simulink model "loop_ctl_flex_test"  (R2019b)
settings: Solver=FixedStepDiscrete  StartTime=0.0  StopTime=400  RelTol=1e-3
libraries: simulink x1, lib_dsphdlcontrol_v1 x1
settings Model: DataTypeOverride=Off  Creator=mbabst  LastModifiedBy=mbabst
settings DataIOCC: SaveOutput=off  SaveTime=off  ReturnWorkspaceOutputs=off
settings OptimizationCC: BlockReduction=off  ConditionallyExecuteInputs=off  DefaultParameterBehavior=Inlined  LifeSpan=inf
settings DebuggingCC: AlgebraicLoopMsg=error  SingleTaskRateTransMsg=error  StrictBusMsg=ErrorOnBusTreatedAsVector  SFUnexpectedBacktrackingDiag=warning  SFNoUnconditionalDefaultTransitionDiag=warning  SFExecutionAtInitializationDiag=none  ArithmeticOperatorsInVariantConditions=warning
settings HardwareCC: ProdBitPerPointer=32  ProdBitPerSizeT=32  ProdBitPerPtrDiffT=32  ProdLargestAtomicFloat=None  ProdIntDivRoundTo=Undefined  ProdEndianess=Unspecified  ProdWordSize=32  ProdHWDeviceType=ASIC/FPGA->ASIC/FPGA  ProdEqTarget=off
settings SFSimCC: SimUseLocalCustomCode=off  CustomCodeUndefinedFunction=UseInterfaceOnly
settings RTWCC: RTWUseLocalCustomCode=off
settings CodeAppCC: StateflowObjectComments=on
settings GRTTargetCC: TargetLangStandard=C89/C90 (ANSI)
settings ConfigComp: CovMetricSettings=dw  CovHtmlReporting=on  CovSaveCumulativeToWorkspaceVar=on  CovSaveSingleToWorkspaceVar=on  CovExternalEMLEnable=off

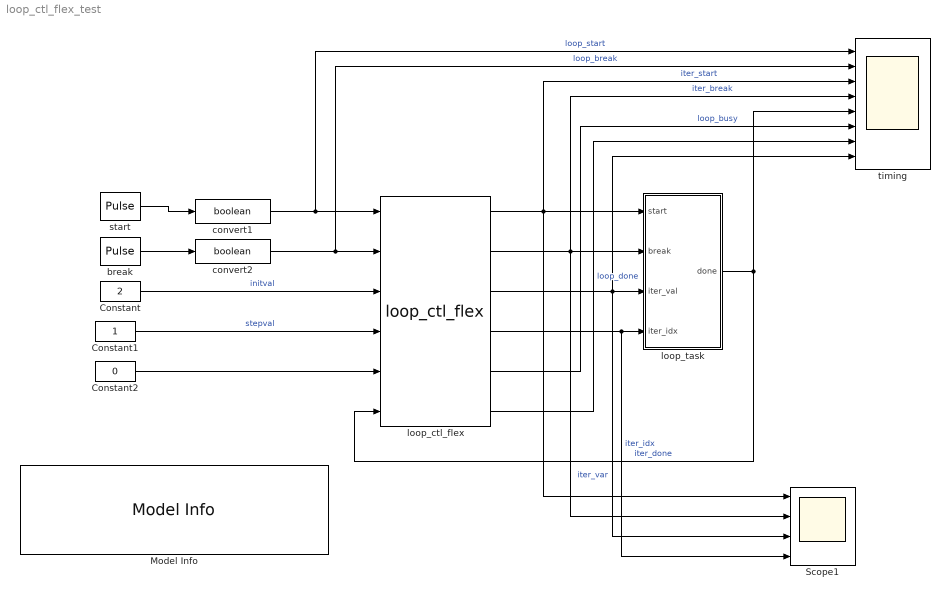
== system loop_ctl_flex_test ==
  Constant : Constant  Value=2  OutDataTypeStr=fixdt(1,8,4)  SampleTime=1
  Constant1 : Constant  OutDataTypeStr=fixdt(1,8,4)  SampleTime=1
  Constant2 : Constant  Value=0  OutDataTypeStr=fixdt(0,3,0)  SampleTime=1
  Model Info : simulink/Model-Wide Utilities/Model Info  Frame=on  DisplayStringWithTags=|  HorizontalTextAlignment=Left  LeftAlignmentValue=0.02
      | Copyright (c) 2005-2021 DSPlogic, Inc.
      | Distributed under the terms of the Simplified BSD License.
      | The full license is in the file LICENSE, distributed with this software.
      | 
      | Model: %<ModelName> (v%<ModelVersion>)
      | Author: Michael Babst <mike.babst@dsplogic.com>
      | Created: by %<Creator> on %<Created>
      | Modified: by %<ModifiedBy> on %<LastModificationDate>
  Scope1 : Scope  NumInputPorts=4
  break : DiscretePulseGenerator  Period=200  PhaseDelay=106
  convert1 : DataTypeConversion  OutDataTypeStr=boolean
  convert2 : DataTypeConversion  OutDataTypeStr=boolean
  loop_ctl_flex : lib_dsphdlcontrol_v1/loop_ctl_flex
      settings: SourceProductName=DSPHDL Library
  loop_task : Subsystem
  start : DiscretePulseGenerator  Period=100  PhaseDelay=5
  timing : Scope  NumInputPorts=8
  wires:
  start/1 -> convert1/1
  Constant/1 -> loop_ctl_flex/3  "initval"
  Constant1/1 -> loop_ctl_flex/4  "stepval"
  loop_task/1(done) -> timing/5, loop_ctl_flex/6  "iter_done"
  convert1/1 -> loop_ctl_flex/1, timing/1  "loop_start"
  Constant2/1 -> loop_ctl_flex/5
  break/1 -> convert2/1
  convert2/1 -> timing/2, loop_ctl_flex/2  "loop_break"
  loop_ctl_flex/2 -> loop_task/2(break), Scope1/2, timing/4  "iter_break"
  loop_ctl_flex/1 -> Scope1/1, timing/3, loop_task/1(start)  "iter_start"
  loop_ctl_flex/3 -> Scope1/3, timing/8, loop_task/3(iter_val)  "iter_var"
  loop_ctl_flex/4 -> Scope1/4, loop_task/4(iter_idx)  "iter_idx"
  loop_ctl_flex/5 -> timing/6  "loop_busy"
  loop_ctl_flex/6 -> timing/7  "loop_done"

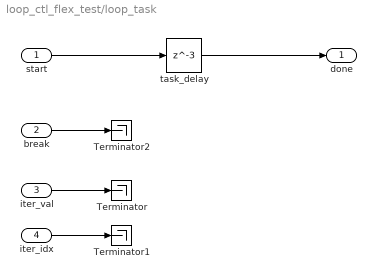
== system loop_ctl_flex_test/loop_task ==
  start : Inport
  break : Inport  Port=2
  iter_val : Inport  Port=3
  iter_idx : Inport  Port=4
  Terminator : Terminator
  Terminator1 : Terminator
  Terminator2 : Terminator
  task_delay : Delay  DelayLength=3  InitialCondition=0
  done : Outport
  wires:
  task_delay/1 -> done/1
  start/1 -> task_delay/1
  iter_val/1 -> Terminator/1
  iter_idx/1 -> Terminator1/1
  break/1 -> Terminator2/1
